simulink model "robust_sliding_mode_control"  (R2021a)
settings: Solver=VariableStepAuto  StartTime=0.0  StopTime=60  RelTol=1e-3
libraries: simulink x1
settings Model: Creator=dell  LastModifiedBy=dell

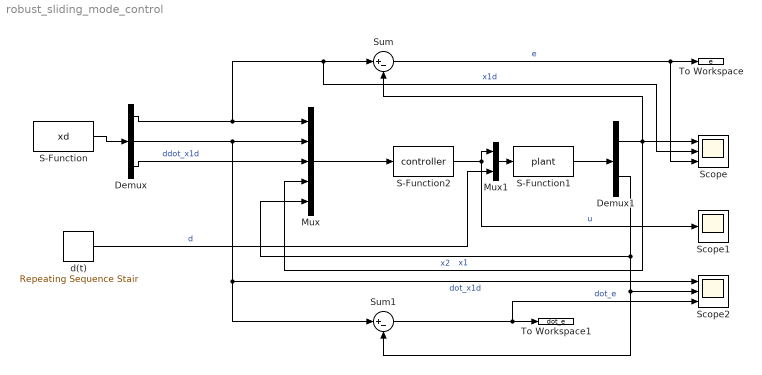
== system robust_sliding_mode_control ==
  Demux : Demux  Outputs=3
  Demux1 : Demux  Outputs=2
  Mux : Mux  Inputs=5
  Mux1 : Mux  Inputs=2
  S-Function : S-Function  FunctionName=xd  Parameters=pa  SFunctionDeploymentMode=off  EnableBusSupport=off
  S-Function1 : S-Function  FunctionName=plant  Parameters=pa  SFunctionDeploymentMode=off  EnableBusSupport=off
  S-Function2 : S-Function  FunctionName=controller  Parameters=pa  SFunctionDeploymentMode=off  EnableBusSupport=off
  Scope : Scope  NumInputPorts=3
  Scope1 : Scope
  Scope2 : Scope  NumInputPorts=3
  Sum : Sum  Inputs=|+-
  Sum1 : Sum  Inputs=|+-
  To Workspace : ToWorkspace  VariableName=e  SampleTime=-1
  To Workspace1 : ToWorkspace  VariableName=dot_e  SampleTime=-1
  d(t) : simulink/Sources/Repeating Sequence Stair  OutValues=[20 22 -20 21 23 15].'  tsamp=10  OutMin=[]  OutMax=[]  OutDataTypeStr=double  OutputDataTypeScalingMode=double  OutDataType=fixdt(0,8)  ConRadixGroup=Best Precision: Vector-wise  OutScaling=2^-12
  wires:
  S-Function/1 -> Demux/1
  Demux/1 -> Scope/2, Sum/1, Mux/1  "x1d"
  Demux/2 -> Sum1/1, Scope2/1, Mux/2  "dot_x1d"
  Demux/3 -> Mux/3  "ddot_x1d"
  S-Function2/1 -> Mux1/1, Scope1/1  "u"
  S-Function1/1 -> Demux1/1
  Demux1/1 -> Scope/1, Sum/2, Mux/4  "x1"
  Demux1/2 -> Scope2/2, Sum1/2, Mux/5  "x2"
  Mux/1 -> S-Function2/1
  Sum/1 -> To Workspace/1, Scope/3  "e"
  Sum1/1 -> To Workspace1/1, Scope2/3  "dot_e"
  Mux1/1 -> S-Function1/1
  d(t)/1 -> Mux1/2  "d"
